simulink model "check_sfunc_nrlmsise00"  (Simulink 7.8)
settings: Solver=ode4  StartTime=0.0  StopTime=10000  FixedStep=0.1  RelTol=1e-3
libraries: aerolibatmos2 x1
settings Model: Creator=kkamiya  LastModifiedBy=kkamiya

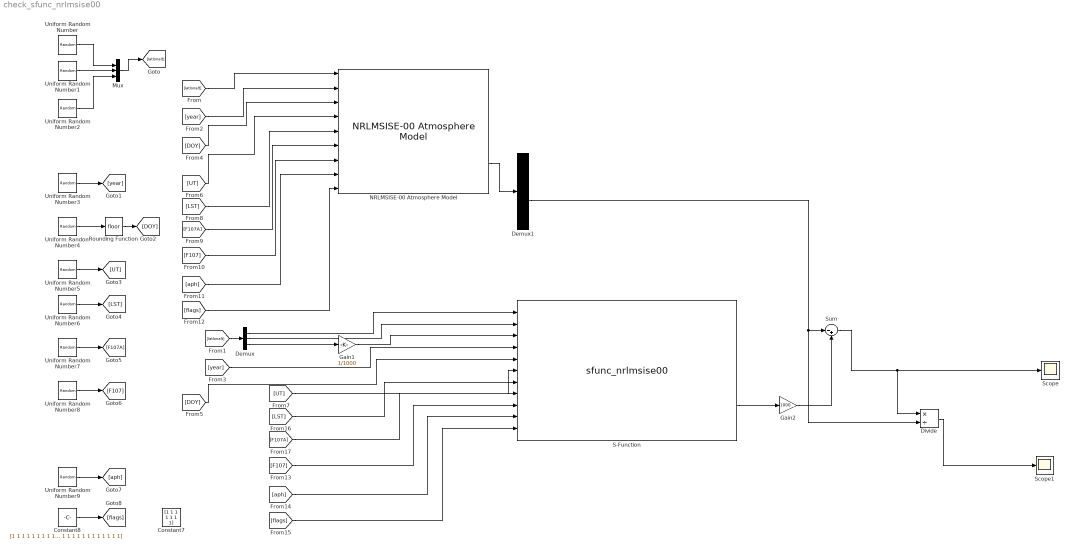
== system check_sfunc_nrlmsise00 ==
  Constant7 : Constant  Value=[1 1 1 1 1 1 1]
  Constant8 : Constant  Value=[1 1 1 1 1 1 1 1 1 1 1 1 1 1 1 1 1 1 1 1 1 1 1]
  Demux : Demux  Outputs=3
  Demux1 : Demux  Outputs=9
  Divide : Product  Inputs=*/
  Gain1 : Gain  Gain=1/1000
  Gain2 : Gain  Gain=1000
  Mux : Mux  Inputs=3
  NRLMSISE-00 Atmosphere Model : aerolibatmos2/NRLMSISE-00 Atmosphere Model  units=Metric (MKS)  lst_input=on  flux_ap_input=on  flags_input=External  flags=ones(1,23)  oxygen_in=off  action=Warning
  Rounding Function : Rounding
  S-Function : S-Function  FunctionName=sfunc_nrlmsise00  EnableBusSupport=off
  Scope : Scope
      settings: YMin=-7e-018  YMax=1.5e-018
  Scope1 : Scope
      settings: YMin=-0.001  YMax=0.0001
  Sum : Sum  Inputs=|-+
  Uniform Random Number : UniformRandomNumber  Minimum=-90  Maximum=90  Seed=-1  SampleTime=0.1
  Uniform Random Number1 : UniformRandomNumber  Minimum=0  Maximum=360  Seed=-2  SampleTime=0.1
  Uniform Random Number2 : UniformRandomNumber  Minimum=300000  Maximum=800000  Seed=-3  SampleTime=0.1
  Uniform Random Number3 : UniformRandomNumber  Minimum=1950  Maximum=2050  Seed=-4  SampleTime=0.1
  Uniform Random Number4 : UniformRandomNumber  Minimum=0  Maximum=365  Seed=-5  SampleTime=0.1
  Uniform Random Number5 : UniformRandomNumber  Minimum=0  Maximum=86400  Seed=-6  SampleTime=0.1
  Uniform Random Number6 : UniformRandomNumber  Minimum=0  Maximum=24  Seed=-7  SampleTime=0.1
  Uniform Random Number7 : UniformRandomNumber  Minimum=1  Maximum=400  Seed=-8  SampleTime=0.1
  Uniform Random Number8 : UniformRandomNumber  Minimum=1  Maximum=400  Seed=-9  SampleTime=0.1
  Uniform Random Number9 : UniformRandomNumber  Minimum=[1 1 1 1 1 1 1]  Maximum=[100 100 100 100 100 100 100]  Seed=[-10 -11 -12 -13 -14 -15 -16]  SampleTime=0.1
  wires:
  Uniform Random Number3/1 -> [year]
  Uniform Random Number5/1 -> [UT]
  Uniform Random Number7/1 -> [F107A]
  Uniform Random Number8/1 -> [F107]
  Constant8/1 -> [flags]
  [latlonalt] -> NRLMSISE-00 Atmosphere Model/1
  [latlonalt] -> Demux/1
  [year] -> NRLMSISE-00 Atmosphere Model/2
  [DOY] -> NRLMSISE-00 Atmosphere Model/3
  [UT] -> NRLMSISE-00 Atmosphere Model/4
  [LST] -> NRLMSISE-00 Atmosphere Model/5
  [F107A] -> NRLMSISE-00 Atmosphere Model/6
  [F107] -> NRLMSISE-00 Atmosphere Model/7
  [aph] -> NRLMSISE-00 Atmosphere Model/8
  [flags] -> NRLMSISE-00 Atmosphere Model/9
  Demux/1 -> S-Function/1
  Demux/2 -> S-Function/2
  Demux/3 -> Gain1/1
  [year] -> S-Function/4
  [DOY] -> S-Function/5
  [UT] -> S-Function/6
  [LST] -> S-Function/7
  [F107A] -> S-Function/8
  [F107] -> S-Function/9
  [aph] -> S-Function/10
  [flags] -> S-Function/11
  S-Function/2 -> Gain2/1
  Gain1/1 -> S-Function/3
  NRLMSISE-00 Atmosphere Model/2 -> Demux1/1
  Demux1/6 -> Sum/1, Divide/2
  Gain2/1 -> Sum/2
  Sum/1 -> Scope/1, Divide/1
  Uniform Random Number/1 -> Mux/1
  Uniform Random Number1/1 -> Mux/2
  Mux/1 -> [latlonalt]
  Uniform Random Number2/1 -> Mux/3
  Uniform Random Number4/1 -> Rounding Function/1
  Uniform Random Number6/1 -> [LST]
  Divide/1 -> Scope1/1
  Uniform Random Number9/1 -> [aph]
  Rounding Function/1 -> [DOY]
